simulink model "DrvDem_SetPoint"  (R2016b)
settings: configuration reference "CodeGenConfigSet" (kept outside this file)
values from neighbouring files (symbols this model uses):
  DrvDem_facDrvSetPPT1_C = Calibration.Parameter    [init_DrvDem_SetPoint.m]    (also in init_DrvDem_SetPoint_SIL.m = Simulink.Parameter)
  DrvDem_nDrvSetPLo_CUR = Calibration.Parameter    [init_DrvDem_SetPoint.m]    (also in init_DrvDem_SetPoint_SIL.m = Simulink.Parameter)
  DrvDem_nDrvSetPLo_CURX = Calibration.Parameter    [init_DrvDem_SetPoint.m]    (also in init_DrvDem_SetPoint_SIL.m = Simulink.Parameter)
  DrvDem_nSpdDem_C = Calibration.Parameter    [init_DrvDem_SetPoint.m]    (also in init_DrvDem_SetPoint_SIL.m = Simulink.Parameter)
  DrvDem_swtDrvNGovActv_C = Calibration.Parameter    [init_DrvDem_SetPoint.m]    (also in init_DrvDem_SetPoint_SIL.m = Simulink.Parameter)
  DrvDem_swtDrvNGovcfg_C = Calibration.Parameter    [init_DrvDem_SetPoint.m]    (also in init_DrvDem_SetPoint_SIL.m = Simulink.Parameter)
  ENG_N_ZERO = fi(0,EngSpeed_rpm)    [init_DrvDem_SetPoint.m]    (also in init_DrvDem_SetPoint_SIL.m)
libraries: simulink x2, CXLib x2
settings Model: Creator=lenovo  LastModifiedBy=xuxingpei
settings ConfigSetRef: SourceLocation=Base Workspace

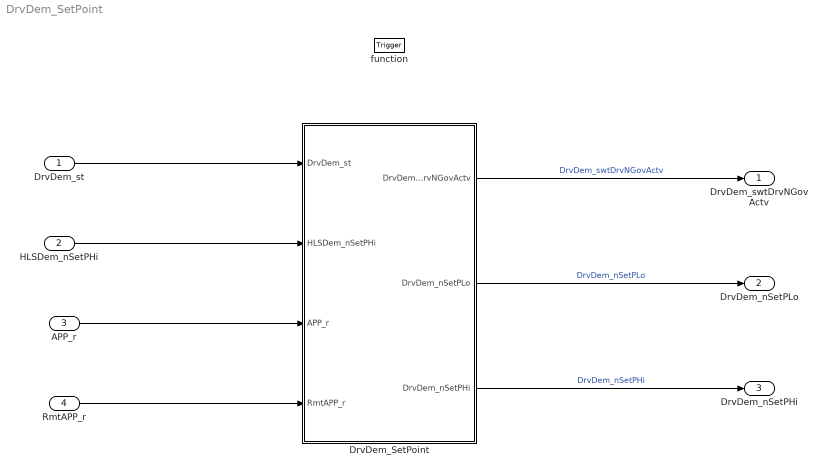
== system DrvDem_SetPoint ==
  DrvDem_st : Inport  Description=Drive demand status to select the pedal for setpoint calculation  OutMin=0  OutMax=255  OutDataTypeStr=State_uint8
  HLSDem_nSetPHi : Inport  Tag=rpm  Description=Maximum engine speed of HLSDem  Port=2  OutMin=0  OutMax=6000  OutDataTypeStr=EngSpeed_rpm
  APP_r : Inport  Tag=%  Description=Acceleration pedal sensor 1 value after fault handling  Port=3  OutMin=0  OutMax=100  OutDataTypeStr=Accpedal_rate
  RmtAPP_r : Inport  Tag=%  Description=Value of Remote accelerator pedal Position  Port=4  OutMin=0  OutMax=100  OutDataTypeStr=Accpedal_rate
  function : TriggerPort  TriggerType=function-call  VariantControl=Variant
  DrvDem_SetPoint : Subsystem
  DrvDem_swtDrvNGovActv : Outport  Description=Switch to activate DrvDem  OutDataTypeStr=Enum: Switch_conv
  DrvDem_nSetPLo : Outport  Tag=rpm  Description=Minimal engine speed of DrvDem  Port=2  OutMin=0  OutMax=6000  OutDataTypeStr=EngSpeed_rpm
  DrvDem_nSetPHi : Outport  Tag=rpm  Description=Maximal engine speed of DrvDem  Port=3  OutMin=0  OutMax=6000  OutDataTypeStr=EngSpeed_rpm
  wires:
  DrvDem_st/1 -> DrvDem_SetPoint/1(DrvDem_st)
  HLSDem_nSetPHi/1 -> DrvDem_SetPoint/2(HLSDem_nSetPHi)
  APP_r/1 -> DrvDem_SetPoint/3(APP_r)
  RmtAPP_r/1 -> DrvDem_SetPoint/4(RmtAPP_r)
  DrvDem_SetPoint/1(DrvDem_swtDrvNGovActv) -> DrvDem_swtDrvNGovActv/1  "DrvDem_swtDrvNGovActv"
  DrvDem_SetPoint/2(DrvDem_nSetPLo) -> DrvDem_nSetPLo/1  "DrvDem_nSetPLo"
  DrvDem_SetPoint/3(DrvDem_nSetPHi) -> DrvDem_nSetPHi/1  "DrvDem_nSetPHi"

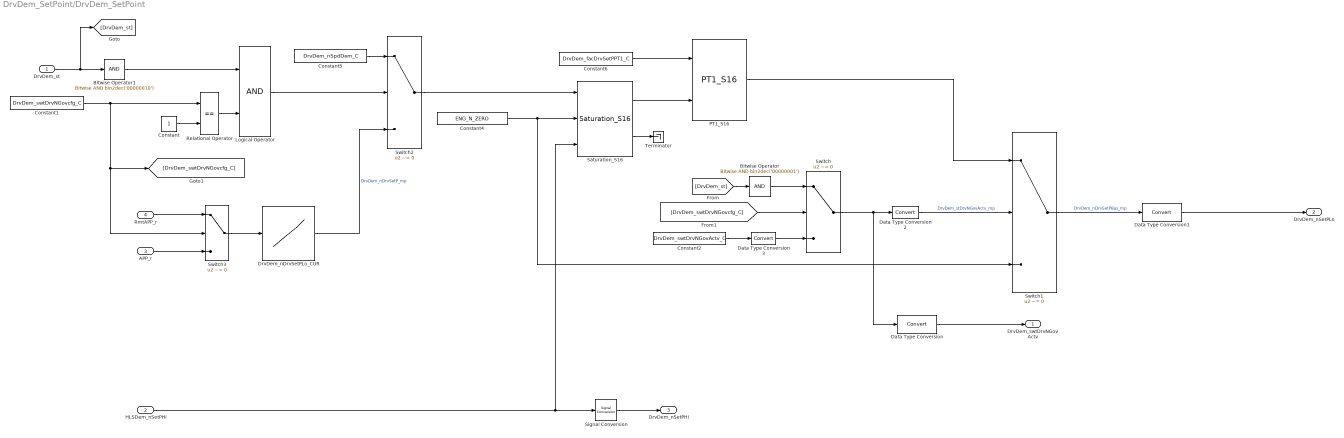
== system DrvDem_SetPoint/DrvDem_SetPoint ==
  DrvDem_st : Inport  Description=Drive demand status to select the pedal for setpoint calculation  OutMin=0  OutMax=255  OutDataTypeStr=State_uint8
  HLSDem_nSetPHi : Inport  Tag=rpm  Description=Maximum engine speed of HLSDem  Port=2  OutMin=0  OutMax=6000  OutDataTypeStr=EngSpeed_rpm
  APP_r : Inport  Tag=%  Description=Acceleration pedal sensor 1 value after fault handling  Port=3  OutMin=0  OutMax=100  OutDataTypeStr=Accpedal_rate
  RmtAPP_r : Inport  Tag=%  Description=Value of Remote accelerator pedal Position  Port=4  OutMin=0  OutMax=100  OutDataTypeStr=Accpedal_rate
  Bitwise Operator : simulink/Logic and Bit Operations/Bitwise Operator  logicop=AND  UseBitMask=on  BitMask=bin2dec('00000001')  BitMaskRealWorld=Stored Integer
  Bitwise Operator1 : simulink/Logic and Bit Operations/Bitwise Operator  logicop=AND  UseBitMask=on  BitMask=bin2dec('00000010')  BitMaskRealWorld=Stored Integer
  Constant : Constant  OutDataTypeStr=Inherit: Inherit via back propagation
  Constant1 : Constant  Value=DrvDem_swtDrvNGovcfg_C
  Constant2 : Constant  Value=DrvDem_swtDrvNGovActv_C
  Constant4 : Constant  Value=ENG_N_ZERO  OutDataTypeStr=Inherit: Inherit via back propagation
  Constant5 : Constant  Value=DrvDem_nSpdDem_C
  Constant6 : Constant  Value=DrvDem_facDrvSetPPT1_C  SampleTime=-1
  Data Type Conversion{,1..3} (4 alike) : DataTypeConversion
  DrvDem_nDrvSetPLo_CUR : Lookup_n-D  NumberOfTableDimensions=1  BreakpointsForDimension1=DrvDem_nDrvSetPLo_CURX  IndexSearchMethod=Linear search  Table=DrvDem_nDrvSetPLo_CUR  ExtrapMethod=Clip  InternalRulePriority=Speed  OutDataTypeStr=Inherit: Inherit via back propagation  RndMeth=Simplest  InputSameDT=on
  Logical Operator : Logic  AllPortsSameDT=off  OutDataTypeStr=boolean
  PT1_S16 : CXLib/PT1_S16
  Relational Operator : RelationalOperator  Operator===  OutDataTypeStr=boolean  RndMeth=Simplest  InputSameDT=on
  Saturation_S16 : CXLib/Saturation_S16
  Signal Conversion : SignalConversion  OverrideOpt=off
  Switch : Switch  Criteria=u2 ~= 0
  Switch1 : Switch  Criteria=u2 ~= 0  InputSameDT=on
  Switch2 : Switch  Criteria=u2 ~= 0
  Switch3 : Switch  Criteria=u2 ~= 0
  Terminator : Terminator
  DrvDem_swtDrvNGovActv : Outport  Description=Switch to activate DrvDem  OutDataTypeStr=Enum: Switch_conv
  DrvDem_nSetPLo : Outport  Tag=rpm  Description=Minimal engine speed of DrvDem  Port=2  OutMin=0  OutMax=6000  OutDataTypeStr=EngSpeed_rpm
  DrvDem_nSetPHi : Outport  Tag=rpm  Description=Maximal engine speed of DrvDem  Port=3  OutMin=0  OutMax=6000  OutDataTypeStr=EngSpeed_rpm
  wires:
  Saturation_S16/2 -> Terminator/1
  APP_r/1 -> Switch3/3
  HLSDem_nSetPHi/1 -> Signal Conversion/1, Saturation_S16/3
  PT1_S16/1 -> Switch1/1
  Saturation_S16/1 -> PT1_S16/2
  DrvDem_nDrvSetPLo_CUR/1 -> Switch2/3  "DrvDem_nDrvSetP_mp"
  Constant6/1 -> PT1_S16/1
  Constant1/1 -> Switch3/2, [DrvDem_swtDrvNGovcfg_C], Relational Operator/1
  Constant4/1 -> Saturation_S16/2, Switch1/3
  Switch2/1 -> Saturation_S16/1
  RmtAPP_r/1 -> Switch3/1
  Switch3/1 -> DrvDem_nDrvSetPLo_CUR/1
  Switch1/1 -> Data Type Conversion1/1  "DrvDem_nDrvSetPBas_mp"
  Data Type Conversion1/1 -> DrvDem_nSetPLo/1
  Data Type Conversion/1 -> DrvDem_swtDrvNGovActv/1
  Signal Conversion/1 -> DrvDem_nSetPHi/1
  Constant/1 -> Relational Operator/2
  Constant5/1 -> Switch2/1
  Data Type Conversion2/1 -> Switch1/2  "DrvDem_stDrvNGovActv_mp"
  Logical Operator/1 -> Switch2/2
  Relational Operator/1 -> Logical Operator/2
  DrvDem_st/1 -> [DrvDem_st], Bitwise Operator1/1
  Bitwise Operator1/1 -> Logical Operator/1
  [DrvDem_st] -> Bitwise Operator/1
  Switch/1 -> Data Type Conversion/1, Data Type Conversion2/1
  Bitwise Operator/1 -> Switch/1
  [DrvDem_swtDrvNGovcfg_C] -> Switch/2
  Constant2/1 -> Data Type Conversion3/1
  Data Type Conversion3/1 -> Switch/3
